simulink model "traj_follower"  (R2022b)
settings: Solver=VariableStepAuto  StartTime=0.0  StopTime=inf  RelTol=1e-3
values from neighbouring files (symbols this model uses):
  traj = planner(map, G, waypoints, 13, 21)    [main.m]    (also in planner.m = [traj; [dx', dy']])
libraries: robotmobilelib x1, robotalgslib x1
settings Model: Creator=amoralesma  LastModifiedBy=amoralesma

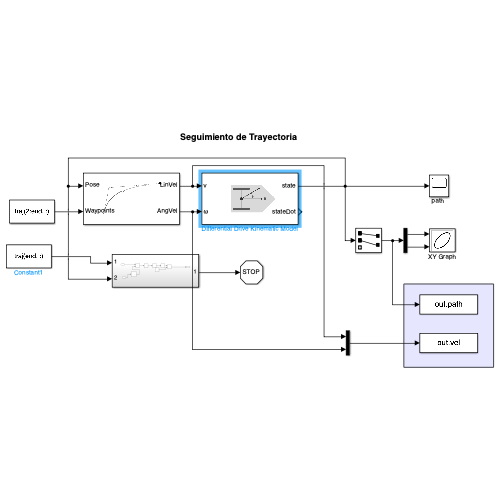
[thumbnail: Simulink's stored preview of the top-level diagram]
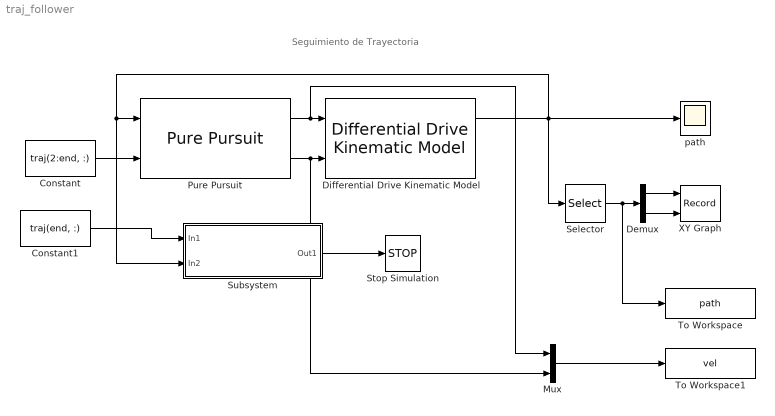
== system traj_follower ==
  note: Seguimiento de Trayectoria
  Constant : Constant  Value=traj(2:end, :)
  Constant1 : Constant  Value=traj(end, :)
  Demux : Demux  Outputs=2
  Differential Drive Kinematic Model : robotmobilelib/Differential Drive Kinematic Model  VehicleInputs=Vehicle Speed & Heading Angular Velocity  WheelRadius=R  WheelSpeedRange=[-inf inf]  TrackWidth=L  InitialState=[traj(2, 1); traj(2, 2); pi/2]  SimulateUsing=Interpreted execution
  Mux : Mux  Inputs=2
  Pure Pursuit : robotalgslib/Pure Pursuit  DesiredLinearVelocity=0.3  MaxAngularVelocity=15.0  LookaheadDistance=0.2  TargetDirPort=off  SimulateUsing=Code generation
      settings: LibrarySourceBlock=robotmobilelib/Pure Pursuit
  Selector : Selector  InputPortWidth=3  IndexOptions=Index vector (dialog)  Indices=[1 2]  OutputSizes=1
  Stop Simulation : Stop
  Subsystem : Subsystem
  To Workspace : ToWorkspace  VariableName=path  SaveFormat=Timeseries  SampleTime=-1
  To Workspace1 : ToWorkspace  VariableName=vel  SaveFormat=Timeseries  SampleTime=-1
  XY Graph : Record  FileSettingsInternal="{\"entries\":[{\"content\":{\"excelSettings\":{\"content\":{},\"type\":\"Streamout.ExcelSettings\"}},\"type\":\"Streamout.FileSettingStorage\",\"uuid\":\"dfdb85b0-ff19-4207-a209-93bdd9bdf03d\"}],\"packageUris\":[\"http://schema.mathworks.com/mf0/streamout_blocks/R2020a\"],\"version\":\"1.0\"}"  Layout=[1 1]  SignalsInternal="{\"entries\":[{\"content\":{\"signals\":[{\"content\":{\"blockPath\":[\"traj_follower/XY Graph\"],\"channel\":[],\"dimensions\":[1],\"domain\":\"traj_follower/XY Graph\",\"lineColor\":\"#a2142f\",\"plots\":[1],\"port\":1,\"sid\":[\"\"],\"signalID\":813,\"signalName\":\"Demux:1\"},\"type\":\"RecordBlkView.Signal\",\"uuid\":\"a6d7b8c7-83fe-4270-bd21-ebf4b7cf30ef\"},{\"content\":{\"blockPath\":[\"traj_follower/XY Graph\"],\"channel\":[],\"dimensions\":[1],\"domain\":\"traj_follower/XY Graph\",\"lineColor\":\"#139fff\",\"plots\":[1],\"port\":2,\"sid\":[\"\"],\"signalID\":817,\"signalName\":\"Demux:2\"},\"type\":\"RecordBlkView.Signal\",\"uuid\":\"acd8dd9d-84a2-49ee-a52a-99696817b492\"}]},\"type\":\"RecordBlkView.InputSignals\",\"uuid\":\"2641d472-55fe-4eba-9200-9abca9ce7827\"}],\"packageUris\":[\"http://schema.mathworks.com/mf0/streamout_blocks/R2020a\"],\"version\":\"1.0\"}"  VisualizationBindings="{\"xyplotplugin\":{\"info\":[{\"series\":[{\"bindingParametersList\":[{\"parameter\":\"X-Axis\",\"signalID\":813,\"signalName\":\"Demux:1\"},{\"parameter\":\"Y-Axis\",\"signalID\":817,\"signalName\":\"Demux:2\"}],\"seriesID\":54294}],\"subplotID\":1}]}}"  CompatibilityTag=XY
  "path " : Scope
  wires:
  Pure Pursuit/1 -> Mux/1, Differential Drive Kinematic Model/1
  Pure Pursuit/2 -> Mux/2, Differential Drive Kinematic Model/2
  Differential Drive Kinematic Model/1 -> Selector/1, "path "/1, Subsystem/2(In2), Pure Pursuit/1
  Constant/1 -> Pure Pursuit/2
  Demux/1 -> XY Graph/1
  Demux/2 -> XY Graph/2
  Selector/1 -> To Workspace/1, Demux/1
  Constant1/1 -> Subsystem/1(In1)
  Subsystem/1(Out1) -> Stop Simulation/1
  Mux/1 -> To Workspace1/1

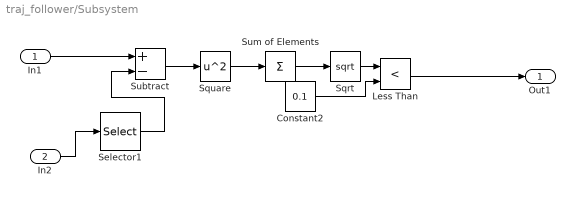
== system traj_follower/Subsystem ==
  In1 : Inport
  In2 : Inport  Port=2
  Constant2 : Constant  Value=0.1
  Less Than : RelationalOperator  Operator=<  OutDataTypeStr=boolean  RndMeth=Simplest  InputSameDT=off
  Selector1 : Selector  InputPortWidth=3  IndexOptions=Index vector (dialog)  Indices=[1 2]  OutputSizes=1
  Sqrt : Sqrt
  Square : Math  Operator=square
  Subtract : Sum  Inputs=+-
  Sum of Elements : Sum  Inputs=+
  Out1 : Outport
  wires:
  In2/1 -> Selector1/1
  Less Than/1 -> Out1/1
  Square/1 -> Sum of Elements/1
  In1/1 -> Subtract/1
  Sum of Elements/1 -> Sqrt/1
  Sqrt/1 -> Less Than/1
  Subtract/1 -> Square/1
  Selector1/1 -> Subtract/2
  Constant2/1 -> Less Than/2
